simulink model "UAV_2010_model_trimming"  (R2023b)
settings: Solver=VariableStepAuto  StartTime=0.0  StopTime=10.0  RelTol=1e-3
settings Model: Creator=aarongreisen  LastModifiedBy=aarongreisen

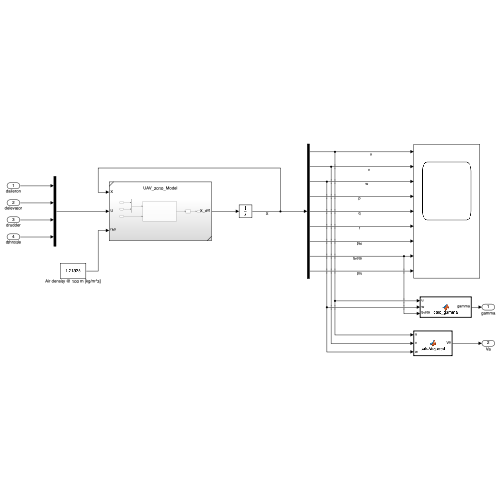
[thumbnail: Simulink's stored preview of the top-level diagram]
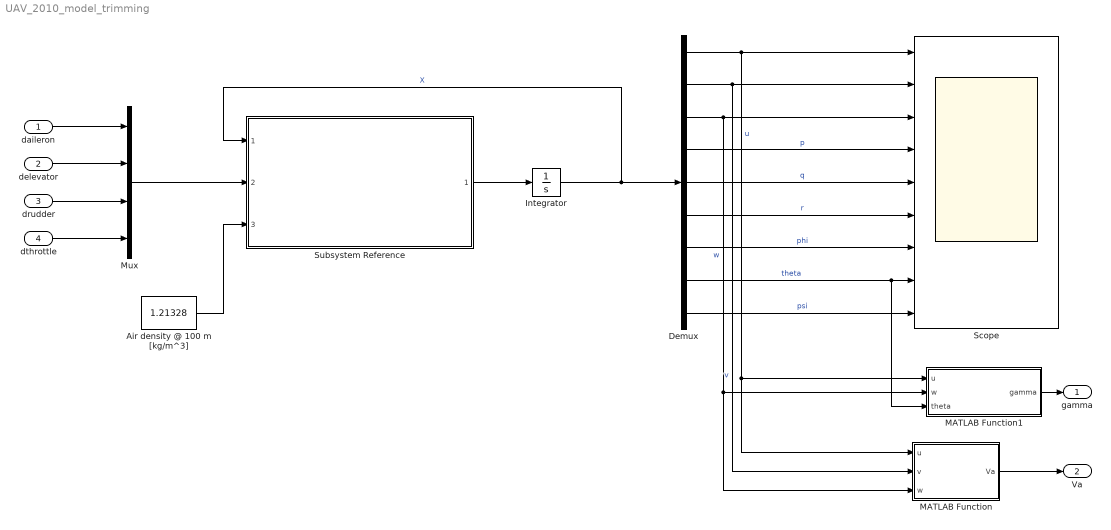
== system UAV_2010_model_trimming ==
  daileron : Inport
  delevator : Inport  Port=2
  drudder : Inport  Port=3
  dthrottle : Inport  Port=4
  Air density @ 100 m [kg/m^3] : Constant  Value=1.21328
  Demux : Demux  Outputs=[1 1 1 1 1 1 1 1 1]
  Integrator : Integrator
  MATLAB Function : MATLAB Function  TreatAsAtomicUnit=on
  MATLAB Function1 : MATLAB Function  TreatAsAtomicUnit=on
  Mux : Mux  Inputs=[1 1 1 1]
  Scope : Scope  NumInputPorts=9
  Subsystem Reference : Subsystem  ReferencedSubsystem=UAV_2010_Model
  gamma : Outport
  Va : Outport  Port=2
  wires:
  Subsystem Reference/1 -> Integrator/1
  Integrator/1 -> Subsystem Reference/1, Demux/1  "X"
  Air density @ 100 m [kg/m^3]/1 -> Subsystem Reference/3
  Mux/1 -> Subsystem Reference/2
  daileron/1 -> Mux/1
  delevator/1 -> Mux/2
  drudder/1 -> Mux/3
  dthrottle/1 -> Mux/4
  Demux/1 -> Scope/1, MATLAB Function1/1(u), MATLAB Function/1(u)  "u"
  Demux/2 -> Scope/2, MATLAB Function/2(v)  "v"
  Demux/3 -> Scope/3, MATLAB Function1/2(w), MATLAB Function/3(w)  "w"
  Demux/4 -> Scope/4  "p"
  Demux/5 -> Scope/5  "q"
  Demux/6 -> Scope/6  "r"
  Demux/7 -> Scope/7  "phi"
  Demux/8 -> MATLAB Function1/3(theta), Scope/8  "theta"
  Demux/9 -> Scope/9  "psi"
  MATLAB Function1/1(gamma) -> gamma/1
  MATLAB Function/1(Va) -> Va/1

== matlab function UAV_2010_model_trimming/MATLAB Function ==
  data: u input; Va output; v input; w input
function Va = calcAirspeed(u, v, w)

Va = sqrt(u^2 + v^2 + w^2);

== matlab function UAV_2010_model_trimming/MATLAB Function1 ==
  data: u input; gamma output; w input; theta input
function gamma = calc_gamma(u, w, theta)

alpha = atan2(w, u);
gamma = theta - alpha;
gamma = rad2deg(gamma);
